simulink model "masks"  (R2019b)
settings: Solver=VariableStepAuto  StartTime=0.0  StopTime=10.0  RelTol=1e-3
settings Model: Creator=bea  LastModifiedBy=bea

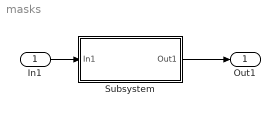
== system masks ==
  In1 : Inport
  Subsystem : Subsystem  mask{g=10}
      mask prompts: g "gain"
  Out1 : Outport
  wires:
  In1/1 -> Subsystem/1(In1)
  Subsystem/1(Out1) -> Out1/1

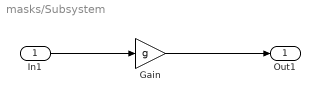
== system masks/Subsystem ==
  In1 : Inport
  "Gain " : Gain  Gain=g
  Out1 : Outport
  wires:
  In1/1 -> "Gain "/1
  "Gain "/1 -> Out1/1
